simulink model "malha_aberta"  (R2019a)
settings: Solver=FixedStepAuto  StartTime=0.0  StopTime=250  FixedStep=.1  RelTol=1e-3
values from neighbouring files (symbols this model uses):
  K = 0.8609    [main.m]
  L = 13.4949    [main.m]
  T = 77.7223    [main.m]
  T_amb = 24.9    [main.m]
settings Model: Creator=paulo  LastModifiedBy=paulo

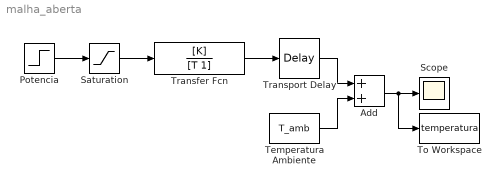
== system malha_aberta ==
  Add : Sum
  Potencia : Step  Time=0  After=30  SampleTime=0
  Saturation : Saturate  UpperLimit=100  LowerLimit=0
  Scope : Scope
  Temperatura Ambiente : Constant  Value=T_amb
  To Workspace : ToWorkspace  VariableName=temperatura  SampleTime=.1
      settings: Save2DSignal=2-D array (concatenate along first dimension)
  Transfer Fcn : TransferFcn  Numerator=[K]  Denominator=[T 1]
  Transport Delay : TransportDelay  DelayTime=L
  wires:
  Saturation/1 -> Transfer Fcn/1
  Potencia/1 -> Saturation/1
  Transfer Fcn/1 -> Transport Delay/1
  Transport Delay/1 -> Add/1
  Add/1 -> To Workspace/1, Scope/1
  Temperatura Ambiente/1 -> Add/2
